simulink model "pool_task"  (Simulink 3.00)
libraries: logiclib x35, mathlib x24, genlib x4, execlib x3, analoglib x2, arclib x2, inoutlib x1

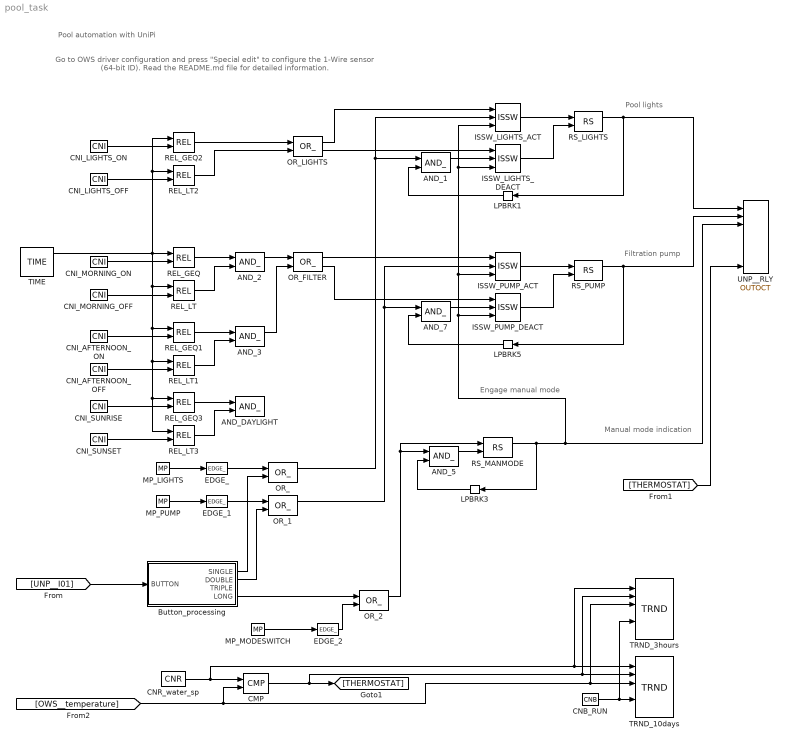
== system pool_task ==
  note: Pool lights
  note: Engage manual mode
  note: Filtration pump
  note: Manual mode indication
  note: Pool automation with UniPi
  note: Go to OWS driver configuration and press "Special edit" to configure the 1-Wire sensor (64-bit ID).
      |
      | Read the README.md file for detailed information.
  AND_{1..3,5,7} (5 alike) : logiclib/AND_
  AND_DAYLIGHT : logiclib/AND_
  Button_processing : Subsystem
      mask Type: REX sequence
  CMP : analoglib/CMP  hys=0.5
  CNB_RUN : mathlib/CNB  YCN=on
  CNI_AFTERNOON_OFF : mathlib/CNI  icn=14
  CNI_AFTERNOON_ON : mathlib/CNI  icn=13
  CNI_LIGHTS_OFF : mathlib/CNI  icn=1
  CNI_LIGHTS_ON : mathlib/CNI  icn=21
  CNI_MORNING_OFF : mathlib/CNI  icn=4
  CNI_MORNING_ON : mathlib/CNI  icn=2
  CNI_SUNRISE : mathlib/CNI  icn=5
  CNI_SUNSET : mathlib/CNI  icn=21
  CNR_water_sp : mathlib/CNR  ycn=26.5
  EDGE_ : logiclib/EDGE_  iedge=1: Rising edge
  EDGE_1 : logiclib/EDGE_  iedge=1: Rising edge
  EDGE_2 : logiclib/EDGE_  iedge=1: Rising edge
  ISSW_LIGHTS_ACT : logiclib/ISSW
  ISSW_LIGHTS_DEACT : logiclib/ISSW
  ISSW_PUMP_ACT : logiclib/ISSW
  ISSW_PUMP_DEACT : logiclib/ISSW
  LPBRK1 : execlib/LPBRK  Orientation=left
  LPBRK3 : execlib/LPBRK  Orientation=left
  LPBRK5 : execlib/LPBRK  Orientation=left
  MP_LIGHTS : genlib/MP  pwidth=0.05  BSTATE=off  RPTF=off
  MP_MODESWITCH : genlib/MP  pwidth=0.05  BSTATE=on  RPTF=off
  MP_PUMP : genlib/MP  pwidth=0.05  BSTATE=off  RPTF=off
  OR_ : logiclib/OR_
  OR_1 : logiclib/OR_
  OR_2 : logiclib/OR_
  OR_FILTER : logiclib/OR_
  OR_LIGHTS : logiclib/OR_
  REL_GEQ{,1..3} (4 alike) : mathlib/REL  irel=6: greater or equal (>=)
  REL_LT{,1..3} (4 alike) : mathlib/REL  irel=3: less than (<)
  RS_LIGHTS : logiclib/RS
  RS_MANMODE : logiclib/RS
  RS_PUMP : logiclib/RS
  TIME : genlib/TIME  tz=1: Local time
  TRND_10days : arclib/TRND  n=4  l=86400  btype=8: Double  ptype1=1: Store  ptype2=1: Store  ptype3=1: Store  ptype4=1: Store  pfac=2000  afac=0  arc=0  id=1  Title=Thermostat actions (10 days)
  TRND_3hours : arclib/TRND  n=4  l=10800  btype=8: Double  ptype1=1: Store  ptype2=1: Store  ptype3=1: Store  ptype4=1: Store  pfac=200  afac=0  arc=0  id=1  Title=Thermostat actions (3 hours)
  UNP__RLY : inoutlib/OUTOCT
  wires:
  AND_1/1 -> ISSW_LIGHTS_DEACT/2
  AND_2/1 -> OR_FILTER/1
  AND_3/1 -> OR_FILTER/2
  AND_5/1 -> RS_MANMODE/2
  AND_7/1 -> ISSW_PUMP_DEACT/2
  Button_processing/1(SINGLE) -> OR_/2
  Button_processing/2(DOUBLE) -> OR_1/2
  Button_processing/4(LONG) -> OR_2/1
  CMP/1 -> [THERMOSTAT], TRND_10days/2, TRND_3hours/2
  CNB_RUN/1 -> TRND_10days/5, TRND_3hours/5
  CNI_AFTERNOON_OFF/1 -> REL_LT1/2
  CNI_AFTERNOON_ON/1 -> REL_GEQ1/2
  CNI_LIGHTS_OFF/1 -> REL_LT2/2
  CNI_LIGHTS_ON/1 -> REL_GEQ2/2
  CNI_MORNING_OFF/1 -> REL_LT/2
  CNI_MORNING_ON/1 -> REL_GEQ/2
  CNI_SUNRISE/1 -> REL_GEQ3/2
  CNI_SUNSET/1 -> REL_LT3/2
  CNR_water_sp/1 -> CMP/1, TRND_10days/1, TRND_3hours/1
  EDGE_/1 -> OR_/1
  EDGE_1/1 -> OR_1/1
  EDGE_2/1 -> OR_2/2
  [UNP__I01] -> Button_processing/1(BUTTON)
  [THERMOSTAT] -> UNP__RLY/8
  [OWS__temperature] -> CMP/2, TRND_10days/3, TRND_3hours/3
  ISSW_LIGHTS_ACT/1 -> RS_LIGHTS/1
  ISSW_LIGHTS_DEACT/1 -> RS_LIGHTS/2
  ISSW_PUMP_ACT/1 -> RS_PUMP/1
  ISSW_PUMP_DEACT/1 -> RS_PUMP/2
  LPBRK1/1 -> AND_1/2
  LPBRK3/1 -> AND_5/2
  LPBRK5/1 -> AND_7/2
  MP_LIGHTS/1 -> EDGE_/1
  MP_MODESWITCH/1 -> EDGE_2/1
  MP_PUMP/1 -> EDGE_1/1
  OR_/1 -> AND_1/1, ISSW_LIGHTS_ACT/2
  OR_1/1 -> AND_7/1, ISSW_PUMP_ACT/2
  OR_2/1 -> AND_5/1, RS_MANMODE/1
  OR_FILTER/1 -> ISSW_PUMP_ACT/1
  OR_FILTER/2 -> ISSW_PUMP_DEACT/1
  OR_LIGHTS/1 -> ISSW_LIGHTS_ACT/1
  OR_LIGHTS/2 -> ISSW_LIGHTS_DEACT/1
  REL_GEQ/1 -> AND_2/1
  REL_GEQ1/1 -> AND_3/1
  REL_GEQ2/1 -> OR_LIGHTS/1
  REL_GEQ3/1 -> AND_DAYLIGHT/1
  REL_LT/1 -> AND_2/2
  REL_LT1/1 -> AND_3/2
  REL_LT2/1 -> OR_LIGHTS/2
  REL_LT3/1 -> AND_DAYLIGHT/2
  RS_LIGHTS/1 -> LPBRK1/1, UNP__RLY/1
  RS_MANMODE/1 -> LPBRK3/1, ISSW_PUMP_DEACT/3, ISSW_PUMP_ACT/3, ISSW_LIGHTS_ACT/3, ISSW_LIGHTS_DEACT/3, UNP__RLY/3
  RS_PUMP/1 -> LPBRK5/1, UNP__RLY/2
  TIME/1 -> REL_GEQ/1, REL_LT/1, REL_GEQ1/1, REL_GEQ3/1, REL_LT3/1, REL_LT1/1, REL_GEQ2/1, REL_LT2/1

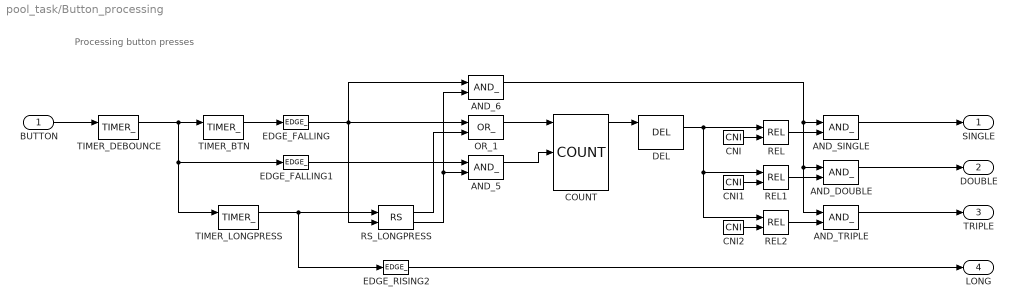
== system pool_task/Button_processing ==
  note: Processing button presses
  BUTTON : Inport  Port=1
  AND_5 : logiclib/AND_
  AND_6 : logiclib/AND_
  AND_DOUBLE : logiclib/AND_
  AND_SINGLE : logiclib/AND_
  AND_TRIPLE : logiclib/AND_
  CNI : mathlib/CNI  icn=1
  CNI1 : mathlib/CNI  icn=2
  CNI2 : mathlib/CNI  icn=3
  COUNT : logiclib/COUNT
  DEL : analoglib/DEL  n=1
  EDGE_FALLING : logiclib/EDGE_  iedge=2: Falling edge
  EDGE_FALLING1 : logiclib/EDGE_  iedge=2: Falling edge
  EDGE_RISING2 : logiclib/EDGE_  iedge=1: Rising edge
  OR_1 : logiclib/OR_
  REL : mathlib/REL  irel=1: equality (==)
  REL1 : mathlib/REL  irel=1: equality (==)
  REL2 : mathlib/REL  irel=1: equality (==)
  RS_LONGPRESS : logiclib/RS
  TIMER_BTN : logiclib/TIMER_  mode=3: Delayed OFF  pt=0.5
  TIMER_DEBOUNCE : logiclib/TIMER_  mode=4: Delayed change  pt=0.01
  TIMER_LONGPRESS : logiclib/TIMER_  mode=2: Delayed ON  pt=3
  SINGLE : Outport  Port=1
  DOUBLE : Outport  Port=2
  TRIPLE : Outport  Port=3
  LONG : Outport  Port=4
  wires:
  AND_5/1 -> COUNT/4
  AND_6/1 -> AND_SINGLE/1, AND_DOUBLE/1, AND_TRIPLE/1
  AND_DOUBLE/1 -> DOUBLE/1
  AND_SINGLE/1 -> SINGLE/1
  AND_TRIPLE/1 -> TRIPLE/1
  BUTTON/1 -> TIMER_DEBOUNCE/1
  CNI/1 -> REL/2
  CNI1/1 -> REL1/2
  CNI2/1 -> REL2/2
  COUNT/1 -> DEL/1
  DEL/1 -> REL/1, REL1/1, REL2/1
  EDGE_FALLING/1 -> AND_6/1, OR_1/1, RS_LONGPRESS/2
  EDGE_FALLING1/1 -> AND_5/1
  EDGE_RISING2/1 -> LONG/1
  OR_1/1 -> COUNT/1
  REL/1 -> AND_SINGLE/2
  REL1/1 -> AND_DOUBLE/2
  REL2/1 -> AND_TRIPLE/2
  RS_LONGPRESS/1 -> OR_1/2
  RS_LONGPRESS/2 -> AND_5/2, AND_6/2
  TIMER_BTN/1 -> EDGE_FALLING/1
  TIMER_DEBOUNCE/1 -> TIMER_BTN/1, EDGE_FALLING1/1, TIMER_LONGPRESS/1
  TIMER_LONGPRESS/1 -> EDGE_RISING2/1, RS_LONGPRESS/1
